simulink model "Buck_Systematic_identification"  (R2023b)
settings: Solver=VariableStepAuto  StartTime=0.0  StopTime=0.01  MaxStep=5e-8  MinStep=1e-8  RelTol=1e-3
libraries: spsSeriesRLCBranchLib x6, spsCurrentMeasurementLib x4, spsMosfetLib x2, spsDCVoltageSourceLib x1, simulink x1, spsVoltageMeasurementLib x1, sps_lib x1
settings Model: Creator=Cr  LastModifiedBy=23227
settings SolverCC: AlgebraicLoopSolver=TrustRegion
settings DataIOCC: ReturnWorkspaceOutputs=off
settings DebuggingCC: UnconnectedInputMsg=warning  UnconnectedOutputMsg=warning  UnconnectedLineMsg=warning  ArithmeticOperatorsInVariantConditions=warning
settings ModelReferenceCC: EnableRefExpFcnMdlSchedulingChecks=on
settings SFSimCC: SimUseLocalCustomCode=off  CustomCodeUndefinedFunction=UseInterfaceOnly
settings RTWCC: RTWUseLocalCustomCode=off
settings CodeAppCC: StateflowObjectComments=on
settings SimscapeCC: SimscapeNormalizeSystem=off

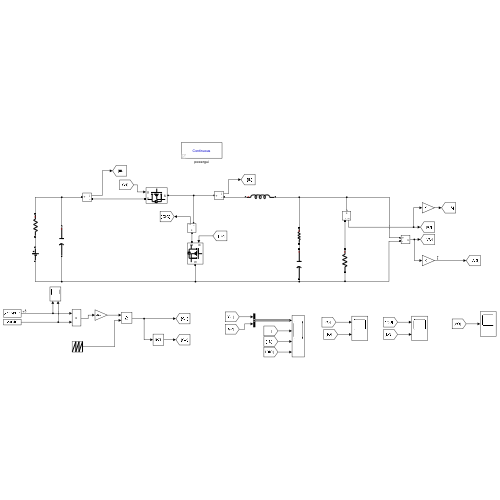
[thumbnail: Simulink's stored preview of the top-level diagram]
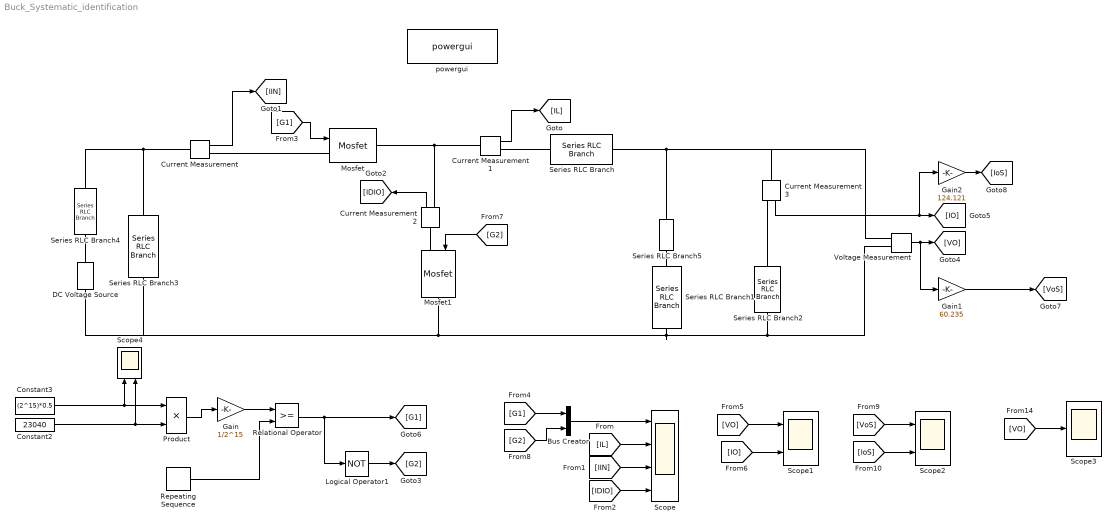
== system Buck_Systematic_identification ==
  Bus Creator : BusCreator  Inputs=2
  Constant2 : Constant  Value=23040
  Constant3 : Constant  Value=(2^15)*0.5
  Current Measurement{,1..3} (4 alike) : spsCurrentMeasurementLib/Current Measurement  PhasorSimulation=off  OutputType=Complex  PSBequivalent=0
  DC Voltage Source : spsDCVoltageSourceLib/DC Voltage Source  Amplitude=48  Measurements=None
  Gain : Gain  Gain=1/2^15
  Gain1 : Gain  Gain=60.235
  Gain2 : Gain  Gain=124.121
  Logical Operator1 : Logic  Operator=NOT  AllPortsSameDT=off  OutDataTypeStr=boolean
  Mosfet : spsMosfetLib/Mosfet  Ron=0.007  Lon=0  Rd=0.01  Vfd=0  IC=0  Rs=1e5  Cs=inf  Measurements=off
  Mosfet1 : spsMosfetLib/Mosfet  Ron=0.007  Lon=0  Rd=0.01  Vfd=0  IC=0  Rs=1e5  Cs=inf  Measurements=off
  Product : Product
  Relational Operator : RelationalOperator  OutDataTypeStr=boolean  RndMeth=Simplest  InputSameDT=off
  Repeating Sequence : simulink/Sources/Repeating Sequence  rep_seq_t=[0 1/200e3]  rep_seq_y=[0 23040]
  Scope : Scope  NumInputPorts=4
  Scope1 : Scope  NumInputPorts=2
  Scope2 : Scope  NumInputPorts=2
  Scope3 : Scope
  Scope4 : Scope  NumInputPorts=2
  Series RLC Branch : spsSeriesRLCBranchLib/Series RLC Branch  LConnTagsString=__new0  RConnTagsString=__new0  BranchType=L  Resistance=1  Inductance=22e-6  SetiL0=off  InitialCurrent=0  Capacitance=1e-6  Setx0=off  InitialVoltage=0  Measurements=None
  Series RLC Branch1 : spsSeriesRLCBranchLib/Series RLC Branch  LConnTagsString=__new0  RConnTagsString=__new0  BranchType=C  Resistance=1  Inductance=1e-3  SetiL0=off  InitialCurrent=0  Capacitance=4.08e-3  Setx0=off  InitialVoltage=0  Measurements=None
  Series RLC Branch2 : spsSeriesRLCBranchLib/Series RLC Branch  LConnTagsString=__new0  RConnTagsString=__new0  BranchType=R  Resistance=2.4  Inductance=1e-3  SetiL0=off  InitialCurrent=0  Capacitance=1e-6  Setx0=off  InitialVoltage=0  Measurements=None
  Series RLC Branch3 : spsSeriesRLCBranchLib/Series RLC Branch  LConnTagsString=__new0  RConnTagsString=__new0  BranchType=C  Resistance=1  Inductance=1e-3  SetiL0=off  InitialCurrent=0  Capacitance=4.08e-3  Setx0=off  InitialVoltage=0  Measurements=None
  Series RLC Branch4 : spsSeriesRLCBranchLib/Series RLC Branch  LConnTagsString=__new0  RConnTagsString=__new0  BranchType=R  Resistance=0.000001  Inductance=1e-3  SetiL0=off  InitialCurrent=0  Capacitance=1e-3  Setx0=off  InitialVoltage=0  Measurements=None
  Series RLC Branch5 : spsSeriesRLCBranchLib/Series RLC Branch  LConnTagsString=__new0  RConnTagsString=__new0  BranchType=R  Resistance=0.033  Inductance=1e-3  SetiL0=off  InitialCurrent=0  Capacitance=1e-6  Setx0=off  InitialVoltage=0  Measurements=None
  Voltage Measurement : spsVoltageMeasurementLib/Voltage Measurement  PhasorSimulation=off  OutputType=Complex  PSBequivalent=0
  powergui : sps_lib/powergui  Priority=1  SimulationMode=Continuous  SampleTime=5e-8  frequency=60  Iterations=50  frequencyindice=0  Pbase=100e6  ErrMax=1e-4  UnitsV=kV  UnitsW=MW  buscounter=0  FunctionMessages=off  echomessages=off  EnableUseOfTLC=off  CurrentSourceSwitches=off  DisableSnubberDevices=off  DisableRonSwitches=off  DisableVfSwitches=off  DisplayEquations=off  AutomaticDiscreteSolvers=off  SolverType=Tustin/Backward Euler (TBE)  Interpol=off  ExternalGateDelay=off  methode=off  Ts=10  x0status=blocks  SPID=off  SwTol=0  HookPort=off  NonlinearTolerance=1e-4  nMaxIteration=100  ContinueOnMaxIteration=off  RestoreLinks=warning  ResistiveCurrentMeasurement=off  Frange=[0:2:500]  Ylog=off  Xlog=on  ShowGrid=off  save=off  variable=ZData  structure=0  ZoomFFT=off  StartTime=0.0  cycles=1  DisplayStyle=1  fundamental=60  FreqAxis=off  MaxFrequency=1000  frequencyindicesteady=1  RmsSteady=1  display=off
  wires:
  Current Measurement1/1 -> [IL]
  [IL] -> Scope/2
  Current Measurement2/1 -> [IDIO]
  [IIN] -> Scope/3
  [IDIO] -> Scope/4
  [G1] -> Mosfet/1
  Voltage Measurement/1 -> Gain1/1, [VO]
  Current Measurement3/1 -> Gain2/1, [IO]
  [VO] -> Scope1/1
  [IO] -> Scope1/2
  [G2] -> Mosfet1/1
  [G1] -> Bus Creator/1
  [G2] -> Bus Creator/2
  Bus Creator/1 -> Scope/1
  Repeating Sequence/1 -> Relational Operator/2
  Relational Operator/1 -> [G1], Logical Operator1/1
  Logical Operator1/1 -> [G2]
  Product/1 -> Gain/1
  Gain/1 -> Relational Operator/1
  Gain1/1 -> [VoS]
  Gain2/1 -> [IoS]
  [IoS] -> Scope2/2
  [VoS] -> Scope2/1
  [VO] -> Scope3/1
  Constant3/1 -> Scope4/1, Product/1
  Constant2/1 -> Product/2, Scope4/2
  Current Measurement/1 -> [IIN]
  connections:
  Current Measurement3/LConn1 -- Voltage Measurement/LConn1 -- Series RLC Branch5/LConn1 -- Series RLC Branch/RConn1
  Series RLC Branch2/RConn1 -- Voltage Measurement/LConn2 -- Series RLC Branch1/RConn1 -- Series RLC Branch3/RConn1 -- DC Voltage Source/LConn1 -- Mosfet1/RConn1
  Series RLC Branch3/LConn1 -- Series RLC Branch4/LConn1 -- Current Measurement/LConn1
  Current Measurement/RConn1 -- Mosfet/LConn1
  Current Measurement1/RConn1 -- Series RLC Branch/LConn1
  Mosfet1/LConn1 -- Current Measurement2/LConn1
  Current Measurement2/RConn1 -- Current Measurement1/LConn1 -- Mosfet/RConn1
  Current Measurement3/RConn1 -- Series RLC Branch2/LConn1
  Series RLC Branch4/RConn1 -- DC Voltage Source/RConn1
  Series RLC Branch5/RConn1 -- Series RLC Branch1/LConn1
